simulink model "Modulador_Torque_equivalente"  (R2023b)
settings: Solver=VariableStepAuto  StartTime=0.0  StopTime=10.0  RelTol=1e-3
values from neighbouring files (symbols this model uses):
  lambda_m = 0.016    [parametros_proyecto2.m]
  Ld = 6.6e-3    (= 0.0066)    [parametros_proyecto2.m]
  Lls = 0.8e-3    (= 0.0008)    [parametros_proyecto2.m]
  Lq = 5.8e-3    (= 0.0058)    [parametros_proyecto2.m]
  r = 120    [parametros_proyecto2.m]
undefined symbols (not defined in the file or in its folder): b_eq, k_l, L_d, L_q, P_p
settings Model: Creator=ignab  LastModifiedBy=ignab

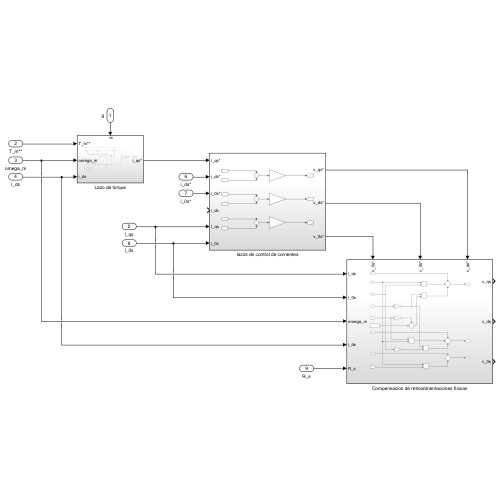
[thumbnail: Simulink's stored preview of the top-level diagram]
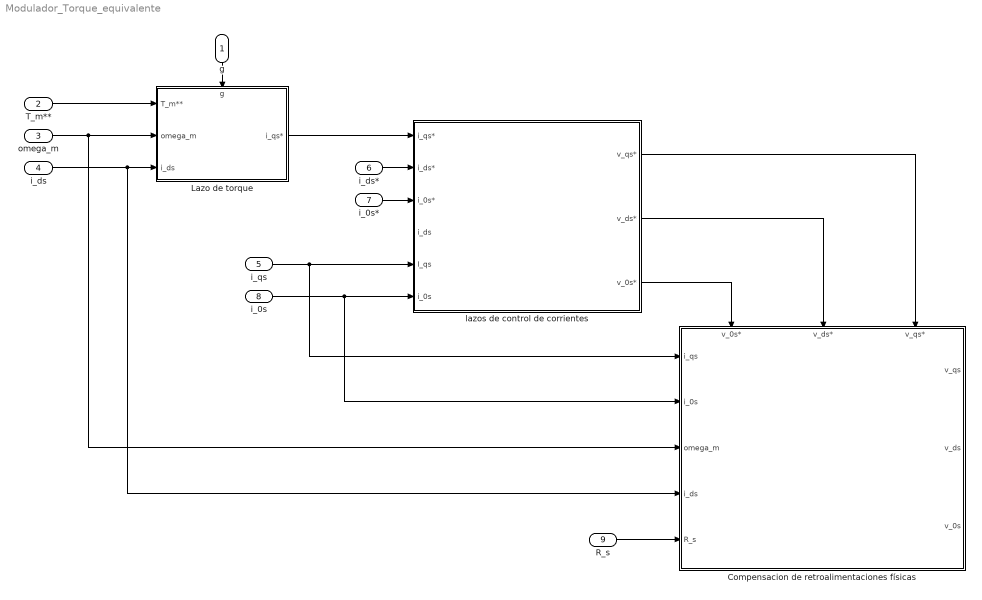
== system Modulador_Torque_equivalente ==
  g : Inport
  T_m** : Inport  Port=2
  omega_m : Inport  Port=3
  i_ds : Inport  Port=4
  i_qs : Inport  Port=5
  i_ds* : Inport  Port=6
  i_0s* : Inport  Port=7
  i_0s : Inport  Port=8
  R_s : Inport  Port=9
  Compensacion de retroalimentaciones físicas : Subsystem
      settings: PortSchema="{\"entries\":[{\"content\":{\"sides\":[{\"content\":{\"connectorIds\":[\"In1\",\"In2\",\"In3\",\"In4\",\"In5\"]},\"type\":\"ConnectorPlacement.EquallySpacedRectSide\",\"uuid\":\"0df91c5b-c04c-40c0-9bfd-240fdb775e59\"},{\"content\":{\"connectorIds\":[\"Out1\",\"Out2\",\"Out3\"],\"side\":\"RIGHT\"},\"type\":\"ConnectorPlacement.EquallySpacedRectSide\",\"uuid\":\"e1c82c1b-ed99-404f-bf55-9e00101b12a7\"},{\"content\":{\"connectorIds\":[\"In6\",\"In7\",\"In8\"],\"side\":\"TOP\"},\"type\":\"ConnectorPlacement.EquallySpacedRectSide\",\"uuid\":\"385ae4cf-1fde-4187-84cf-f7649c337d1a\"}]},\"type\":\"ConnectorPlacement.EquallySpacedConnector\",\"uuid\":\"2ad1d1a3-258a-4dd6-ae6f-3c458114becf\"}],\"packageUris\":[\"http://schema.mathworks.com/mf0/Connector/R2020b\"],\"version\":\"1.0\"}"
  Lazo de torque : Subsystem
      settings: PortSchema="{\"entries\":[{\"content\":{\"sides\":[{\"content\":{\"connectorIds\":[\"In1\",\"In2\",\"In3\"]},\"type\":\"ConnectorPlacement.EquallySpacedRectSide\",\"uuid\":\"d90e2df1-11e0-4ad0-a285-1dd5e4eb856e\"},{\"content\":{\"connectorIds\":[\"Out1\"],\"side\":\"RIGHT\"},\"type\":\"ConnectorPlacement.EquallySpacedRectSide\",\"uuid\":\"59dc5253-0f48-4c82-9c1c-081b0d94a9d5\"},{\"content\":{\"connectorIds\":[\"In4\"],\"side\":\"TOP\"},\"type\":\"ConnectorPlacement.EquallySpacedRectSide\",\"uuid\":\"84f51de4-2005-4450-b7b2-285911307ca8\"}]},\"type\":\"ConnectorPlacement.EquallySpacedConnector\",\"uuid\":\"e7b3a63d-e685-48db-8f20-d049856f721c\"}],\"packageUris\":[\"http://schema.mathworks.com/mf0/Connector/R2020b\"],\"version\":\"1.0\"}"
  lazos de control de corrientes : Subsystem
  wires:
  Lazo de torque/1(i_qs*) -> lazos de control de corrientes/1(i_qs*)
  lazos de control de corrientes/1(v_qs*) -> Compensacion de retroalimentaciones físicas/8(v_qs*)
  lazos de control de corrientes/2(v_ds*) -> Compensacion de retroalimentaciones físicas/7(v_ds*)
  lazos de control de corrientes/3(v_0s*) -> Compensacion de retroalimentaciones físicas/6(v_0s*)
  g/1 -> Lazo de torque/4(g)
  T_m**/1 -> Lazo de torque/1(T_m**)
  omega_m/1 -> Compensacion de retroalimentaciones físicas/3(omega_m), Lazo de torque/2(omega_m)
  i_ds/1 -> Compensacion de retroalimentaciones físicas/4(i_ds), Lazo de torque/3(i_ds)
  i_qs/1 -> Compensacion de retroalimentaciones físicas/1(i_qs), lazos de control de corrientes/5(I_qs)
  i_ds*/1 -> lazos de control de corrientes/2(i_ds*)
  i_0s*/1 -> lazos de control de corrientes/3(i_0s*)
  i_0s/1 -> Compensacion de retroalimentaciones físicas/2(i_0s), lazos de control de corrientes/6(i_0s)
  R_s/1 -> Compensacion de retroalimentaciones físicas/5(R_s)

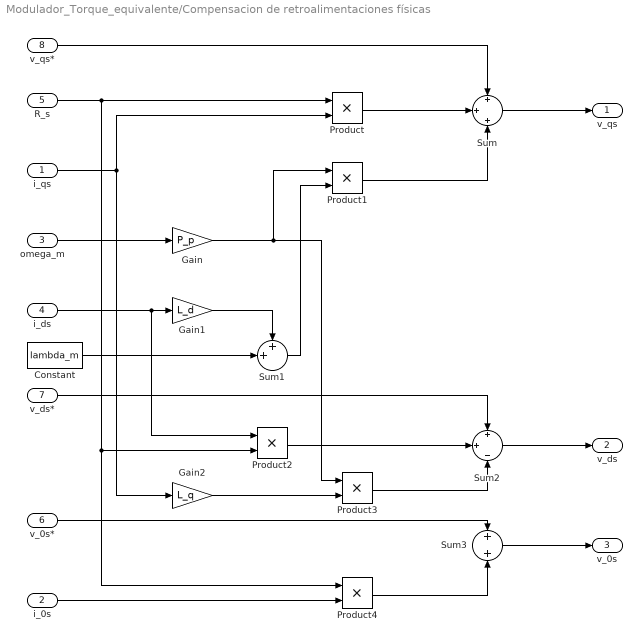
== system Modulador_Torque_equivalente/Compensacion de retroalimentaciones físicas ==
  i_qs : Inport
  i_0s : Inport  Port=2
  omega_m : Inport  Port=3
  i_ds : Inport  Port=4
  R_s : Inport  Port=5
  v_0s* : Inport  Port=6
  v_ds* : Inport  Port=7
  v_qs* : Inport  Port=8
  Constant : Constant  Value=lambda_m
  Gain : Gain  Gain=P_p
  Gain1 : Gain  Gain=L_d
  Gain2 : Gain  Gain=L_q
  Product{,1..4} (5 alike) : Product
  Sum : Sum  Inputs=+|+|+
  Sum1 : Sum  Inputs=++|
  Sum2 : Sum  Inputs=+|+|-
  Sum3 : Sum  Inputs=+|+
  v_qs : Outport
  v_ds : Outport  Port=2
  v_0s : Outport  Port=3
  wires:
  Gain2/1 -> Product3/2
  Sum1/1 -> Product1/2
  Gain/1 -> Product3/1, Product1/1
  omega_m/1 -> Gain/1
  R_s/1 -> Product4/1, Product2/2, Product/1
  Product1/1 -> Sum/3
  Product/1 -> Sum/2
  Sum2/1 -> v_ds/1
  i_0s/1 -> Product4/2
  Gain1/1 -> Sum1/1
  Product4/1 -> Sum3/2
  Sum3/1 -> v_0s/1
  Sum/1 -> v_qs/1
  v_qs*/1 -> Sum/1
  v_ds*/1 -> Sum2/1
  v_0s*/1 -> Sum3/1
  Constant/1 -> Sum1/2
  Product2/1 -> Sum2/2
  Product3/1 -> Sum2/3
  i_ds/1 -> Product2/1, Gain1/1
  i_qs/1 -> Gain2/1, Product/2

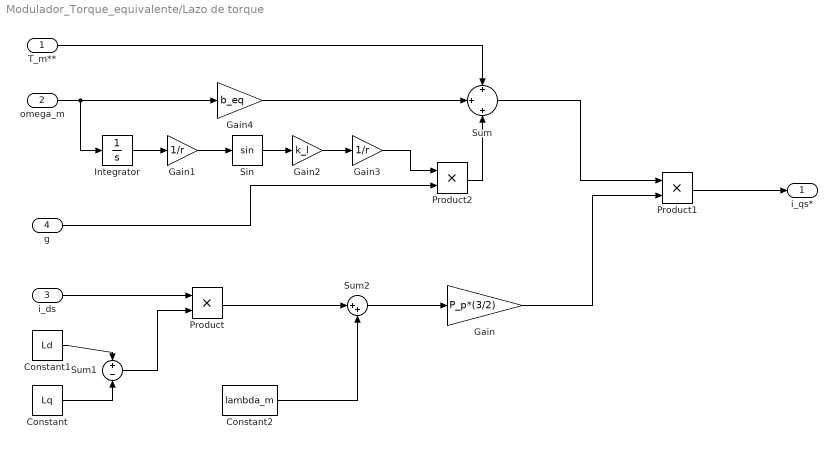
== system Modulador_Torque_equivalente/Lazo de torque ==
  T_m** : Inport
  omega_m : Inport  Port=2
  i_ds : Inport  Port=3
  g : Inport  Port=4
  Constant : Constant  Value=Lq
  Constant1 : Constant  Value=Ld
  Constant2 : Constant  Value=lambda_m
  Gain : Gain  Gain=P_p*(3/2)
  Gain1 : Gain  Gain=1/r
  Gain2 : Gain  Gain=k_l
  Gain3 : Gain  Gain=1/r
  Gain4 : Gain  Gain=b_eq
  Integrator : Integrator
  Product : Product
  Product1 : Product
  Product2 : Product
  Sin : Trigonometry
  Sum : Sum  Inputs=+|+|+
  Sum1 : Sum  Inputs=+|-
  Sum2 : Sum  Inputs=|++
  i_qs* : Outport
  wires:
  Constant/1 -> Sum1/2
  Gain4/1 -> Sum/2
  T_m**/1 -> Sum/1
  Sin/1 -> Gain2/1
  omega_m/1 -> Integrator/1, Gain4/1
  Sum1/1 -> Product/2
  Gain/1 -> Product1/2
  Gain1/1 -> Sin/1
  Product/1 -> Sum2/1
  Product2/1 -> Sum/3
  Sum/1 -> Product1/1
  Product1/1 -> i_qs*/1
  Sum2/1 -> Gain/1
  Gain3/1 -> Product2/1
  Gain2/1 -> Gain3/1
  Constant2/1 -> Sum2/2
  Integrator/1 -> Gain1/1
  i_ds/1 -> Product/1
  g/1 -> Product2/2
  Constant1/1 -> Sum1/1

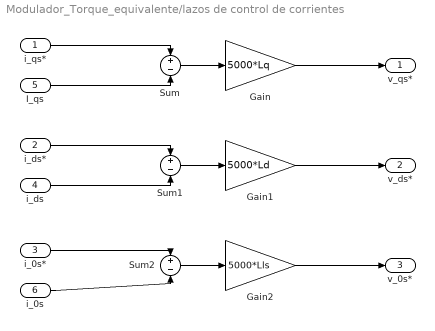
== system Modulador_Torque_equivalente/lazos de control de corrientes ==
  i_qs* : Inport
  i_ds* : Inport  Port=2
  i_0s* : Inport  Port=3
  i_ds : Inport  Port=4
  I_qs : Inport  Port=5
  i_0s : Inport  Port=6
  Gain : Gain  Gain=5000*Lq
  Gain1 : Gain  Gain=5000*Ld
  Gain2 : Gain  Gain=5000*Lls
  Sum : Sum  Inputs=+|-
  Sum1 : Sum  Inputs=+|-
  Sum2 : Sum  Inputs=+|-
  v_qs* : Outport
  v_ds* : Outport  Port=2
  v_0s* : Outport  Port=3
  wires:
  Gain2/1 -> v_0s*/1
  i_0s/1 -> Sum2/2
  i_ds/1 -> Sum1/2
  i_qs*/1 -> Sum/1
  Sum2/1 -> Gain2/1
  Sum1/1 -> Gain1/1
  i_0s*/1 -> Sum2/1
  i_ds*/1 -> Sum1/1
  Sum/1 -> Gain/1
  Gain1/1 -> v_ds*/1
  I_qs/1 -> Sum/2
  Gain/1 -> v_qs*/1
